simulink model "Power_electronics_basic_simulation"  (R2013a)
settings: Solver=FixedStepDiscrete  SolverMode=SingleTasking  StartTime=0.0  StopTime=0.1  MaxStep=Ts  RelTol=1e-3
InitFcn:
  | Ts=1/60/3240;
libraries: powerlib x22, powerlib_extras x2
Description:
  | Copyright 2008-2013 The MathWorks, Inc.
settings Model: ExtModeTrigMode=oneshot  ExtModeArmWhenConnect=off  ExtModeAutoUpdateStatusClock=off  Creator=MathWorks  LastModifiedBy=user
settings DataIOCC: LimitDataPoints=off  SignalLoggingSaveFormat=ModelDataLogs  SignalLoggingName=sigsOut
settings OptimizationCC: BlockReduction=off  BooleanDataType=off  ExpressionDepthLimit=2147483647  InitFltsAndDblsToZero=on  EfficientMapNaN2IntZero=off
settings DebuggingCC: SaveWithParameterizedLinksMsg=none  CheckExecutionContextPreStartOutputMsg=on  CheckExecutionContextRuntimeOutputMsg=on  SignalResolutionControl=TryResolveAllWithWarning  SolverPrmCheckMsg=none  MultiTaskDSMMsg=warning  MultiTaskCondExecSysMsg=none  FcnCallInpInsideContextMsg=UseLocalSettings
settings HardwareCC: TargetUnknown=on
settings RTWCC: IncludeERTFirstTime=on
settings GRTTargetCC: TargetFcnLib=ansi_tfl_tmw.mat  CombineOutputUpdateFcns=off  GRTInterface=on

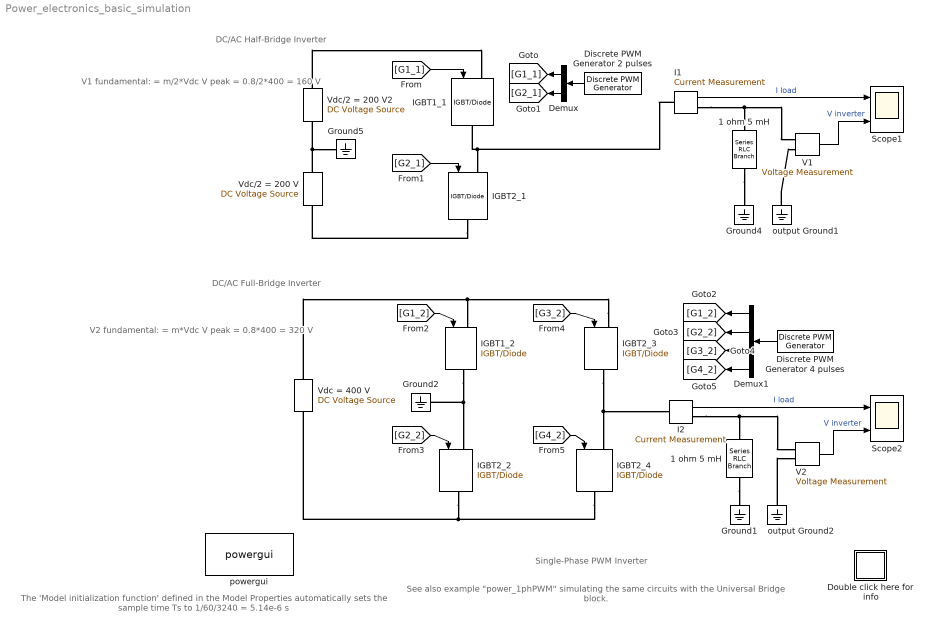
== system Power_electronics_basic_simulation ==
  note: The 'Model  initialization function' defined in the
      | Model Properties automatically sets the sample time Ts
      | to 1/60/3240 = 5.14e-6 s
  note: V1 fundamental:
      |     = m/2*Vdc V peak
      |     = 0.8/2*400
      |     = 160 V
  note: DC/AC Half-Bridge Inverter
  note: DC/AC Full-Bridge Inverter
  note: V2 fundamental:
      |     = m*Vdc V peak
      |     = 0.8*400
      |     = 320 V
  note: Single-Phase PWM Inverter
  note: See also example "power_1phPWM" simulating
      | the same circuits with the Universal Bridge block.
  1 ohm 5 mH : powerlib/Elements/Series RLC Branch  LConnTagsString=__new0  RConnTagsString=__new0  BranchType=RL  Resistance=1  Inductance=5e-03  SetiL0=off  InitialCurrent=0  Capacitance=[]  Setx0=off  InitialVoltage=0  Measurements=None
  "1 ohm 5 mH " : powerlib/Elements/Series RLC Branch  LConnTagsString=__new0  RConnTagsString=__new0  BranchType=RL  Resistance=1  Inductance=5e-03  SetiL0=off  InitialCurrent=0  Capacitance=[]  Setx0=off  InitialVoltage=0  Measurements=None
  Demux : Demux  Outputs=2
  Demux1 : Demux
  Discrete PWM Generator 2 pulses : powerlib_extras/Discrete  Control Blocks/Discrete PWM Generator  GeneratorMode="1-arm  bridge (2 pulses)"  Fc=2000  Ts=Ts  Internal=on  mIndex=0.8  Freq=60  Phase=0
  Discrete PWM Generator 4 pulses : powerlib_extras/Discrete  Control Blocks/Discrete PWM Generator  GeneratorMode="2-arm  bridge (4 pulses)"  Fc=2000  Ts=Ts  Internal=on  mIndex=0.8  Freq=60  Phase=0
  Double click here for info : Subsystem
      settings: OpenFcn=showdemo(bdroot(gcb))
      mask Display: disp('?')
  Ground{1..2,4..5} (4 alike) : powerlib/Elements/Ground  LConnTagsString=a
  I1 : powerlib/Measurements/Current Measurement  Tag=PoWeRsYsTeMmEaSuReMeNt  PhasorSimulation=off  OutputType=Magnitude  PSBequivalent=0
  I2 : powerlib/Measurements/Current Measurement  Tag=PoWeRsYsTeMmEaSuReMeNt  PhasorSimulation=off  OutputType=Magnitude  PSBequivalent=0
  IGBT1_1 : powerlib/Power Electronics/IGBT//Diode  Ron=1e-3  Rs=1e5  Cs=inf  Measurements=off
  IGBT1_2 : powerlib/Power Electronics/IGBT//Diode  Ron=1e-3  Rs=1e5  Cs=inf  Measurements=off
  IGBT2_{1..4} (4 alike) : powerlib/Power Electronics/IGBT//Diode  Ron=1e-3  Rs=1e5  Cs=inf  Measurements=off
  Scope1 : Scope  NumInputPorts=2
      settings: TimeRange=0.1  YMin=-100~-300  YMax=100~300  SaveName=sps1phPWM1_str  MaxDataPoints=500000
  Scope2 : Scope  NumInputPorts=2
      settings: TimeRange=0.1  YMin=-200~-500  YMax=200~500  SaveName=sps1phPWM2_str  MaxDataPoints=500000
  V1 : powerlib/Measurements/Voltage Measurement  Tag=PoWeRsYsTeMmEaSuReMeNt  PhasorSimulation=off  OutputType=Magnitude  PSBequivalent=0
  V2 : powerlib/Measurements/Voltage Measurement  Tag=PoWeRsYsTeMmEaSuReMeNt  PhasorSimulation=off  OutputType=Magnitude  PSBequivalent=0
  Vdc = 400 V : powerlib/Electrical Sources/DC Voltage Source  Description=source block  Amplitude=400  Measurements=None
      settings: AttributesFormatString=\n
  Vdc/2 = 200 V : powerlib/Electrical Sources/DC Voltage Source  Description=source block  Amplitude=200  Measurements=None
      settings: AttributesFormatString=\n
  Vdc/2 = 200 V2 : powerlib/Electrical Sources/DC Voltage Source  Description=source block  Amplitude=200  Measurements=None
      settings: AttributesFormatString=\n
  output Ground1 : powerlib/Elements/Ground  LConnTagsString=a
  output Ground2 : powerlib/Elements/Ground  LConnTagsString=a
  powergui : powerlib/powergui  SimulationMode=Discrete  SolverType=Tustin  SampleTime=Ts  frequency=60  SPID=off  DisableSnubberDevices=off  DisableRonSwitches=off  DisableVfSwitches=off  SwTol=0  Interpol=off  DisplayEquations=off  frequencyindice=0  Pbase=100e6  ErrMax=1e-4  Iterations=50  UnitsV=kV  UnitsW=MW  FunctionMessages=off  echomessages=off  HookPort=off  EnableUseOfTLC=off  x0status=blocks  RestoreLinks=warning  ResistiveCurrentMeasurement=off  Frange=[0:2:500]  Ylog=off  Xlog=on  ShowGrid=off  save=off  variable=ZData  structure=sps1phPWM1_str  ZoomFFT=off  StartTime=0.1-2/60  cycles=2  DisplayStyle=1  fundamental=60  FreqAxis=off  MaxFrequency=5000  frequencyindicesteady=1  RmsSteady=1  display=off  Ts=0  methode=off
  wires:
  I1/1 -> Scope1/1  "I load"
  V1/1 -> Scope1/2  "V inverter"
  Discrete PWM Generator 2 pulses/1 -> Demux/1
  Demux/1 -> [G1_1]
  Demux/2 -> [G2_1]
  [G1_1] -> IGBT1_1/1
  [G2_1] -> IGBT2_1/1
  I2/1 -> Scope2/1  "I load"
  V2/1 -> Scope2/2  "V inverter"
  Discrete PWM Generator 4 pulses/1 -> Demux1/1
  Demux1/1 -> [G1_2]
  Demux1/2 -> [G2_2]
  [G1_2] -> IGBT1_2/1
  [G2_2] -> IGBT2_2/1
  Demux1/3 -> [G3_2]
  Demux1/4 -> [G4_2]
  [G3_2] -> IGBT2_3/1
  [G4_2] -> IGBT2_4/1
  connections:
  I1/RConn1 -- V1/LConn1 -- 1 ohm 5 mH/LConn1
  Vdc/2 = 200 V/RConn1 -- Ground5/LConn1 -- Vdc/2 = 200 V2/LConn1
  1 ohm 5 mH/RConn1 -- Ground4/LConn1
  output Ground1/LConn1 -- V1/LConn2
  IGBT2_1/RConn1 -- Vdc/2 = 200 V/LConn1
  Vdc/2 = 200 V2/RConn1 -- IGBT1_1/LConn1
  I2/RConn1 -- "1 ohm 5 mH "/LConn1 -- V2/LConn1
  "1 ohm 5 mH "/RConn1 -- Ground1/LConn1
  output Ground2/LConn1 -- V2/LConn2
  IGBT2_4/RConn1 -- Vdc = 400 V/LConn1 -- IGBT2_2/RConn1
  IGBT2_3/LConn1 -- Vdc = 400 V/RConn1 -- IGBT1_2/LConn1
  I1/LConn1 -- IGBT1_1/RConn1 -- IGBT2_1/LConn1
  IGBT1_2/RConn1 -- IGBT2_2/LConn1 -- Ground2/LConn1
  IGBT2_3/RConn1 -- IGBT2_4/LConn1 -- I2/LConn1

== system Power_electronics_basic_simulation/Double click here for info ==
